simulink model "electric_motor_no_inductance"  (R2016b)
settings: Solver=FixedStepAuto  StartTime=0.0  StopTime=10.0  FixedStep=0.001  RelTol=1e-3
values from neighbouring files (symbols this model uses):
  b = 0.0192651860035    [exp12_params.mat]    (also in exp14_params.mat = 0.103947574287; motor_calculated_parameters.mat = 0.0173555097)
  beta = 0.000833794079942    [exp12_params.mat]    (also in exp14_params.mat = 5.14977821893e-05; motor_calculated_parameters.mat = 0.000149678)
  J = 0.00104657206588    [exp12_params.mat]    (also in exp14_params.mat = 0.00135; motor_calculated_parameters.mat = 0.00123078313678)
  K = 0.196211074092    [exp12_params.mat]    (also in exp14_params.mat = 0.1881; motor_calculated_parameters.mat = 0.195657531547)
  R = 2.24976937182    [exp12_params.mat]    (also in exp14_params.mat = 1.85035542466; motor_calculated_parameters.mat = 2.39)
settings Model: Creator=piotr  LastModifiedBy=piotr

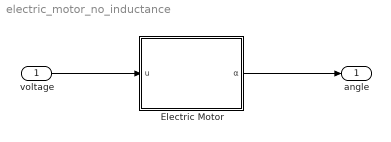
== system electric_motor_no_inductance ==
  voltage : Inport
  Electric Motor : Subsystem  mask{K=K, R=R, beta=beta, b=b, J=J}
      mask prompts: K "Motor constant"; R "Electrical resistance [Ω]"; beta "Motor viscous damping [N*m*s/rad]"; b "Motor dry damping [N*m]"; J "Motor moment of inertia [kg*m^2]"
  angle : Outport
  wires:
  voltage/1 -> Electric Motor/1(u)
  Electric Motor/1(α) -> angle/1

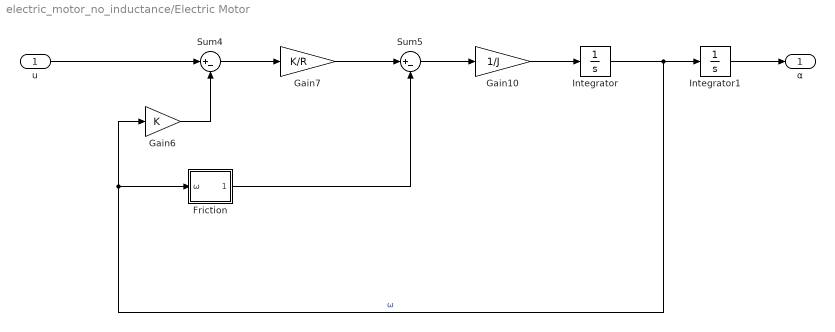
== system electric_motor_no_inductance/Electric Motor ==
  u : Inport
  Friction : Subsystem
  Gain10 : Gain  Gain=1/J
  Gain6 : Gain  Gain=K
  Gain7 : Gain  Gain=K/R
  Integrator : Integrator
  Integrator1 : Integrator
  Sum4 : Sum  Inputs=|+-
  Sum5 : Sum  Inputs=|+-
  α : Outport
  wires:
  Integrator/1 -> Integrator1/1, Gain6/1, Friction/1(ω)  "ω"
  u/1 -> Sum4/1
  Gain6/1 -> Sum4/2
  Sum4/1 -> Gain7/1
  Gain7/1 -> Sum5/1
  Sum5/1 -> Gain10/1
  Gain10/1 -> Integrator/1
  Integrator1/1 -> α/1
  Friction/1(Out1) -> Sum5/2

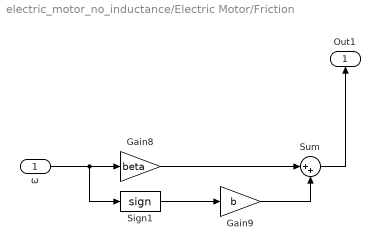
== system electric_motor_no_inductance/Electric Motor/Friction ==
  ω : Inport
  Gain8 : Gain  Gain=beta
  Gain9 : Gain  Gain=b
  Sign1 : Signum  ZeroCross=off
  Sum : Sum  Inputs=|++
  Out1 : Outport
  wires:
  ω/1 -> Sign1/1, Gain8/1
  Sign1/1 -> Gain9/1
  Gain8/1 -> Sum/1
  Sum/1 -> Out1/1
  Gain9/1 -> Sum/2
